simulink model "SOFC_smlkH2"  (R2015b)
settings: Solver=ode113  SolverMode=SingleTasking  StartTime=0.0  StopTime=1000  MaxStep=1  MinStep=0.00001  RelTol=1e-3
values from neighbouring files (symbols this model uses):
  A_an = 1.05e-05    [SOFC_CH4data.m]    (also in SOFC_H2data.m)
  A_cat = 2.38e-05    [SOFC_CH4data.m]    (also in SOFC_H2data.m)
  A_cell = 180    [SOFC_begin.m]
  A_el = 0.03 / T    [SOFC_CH4data.m]    (also in SOFC_H2data.m)
  B_an = -1150    [SOFC_CH4data.m]    (also in SOFC_H2data.m)
  B_cat = 1200    [SOFC_CH4data.m]    (also in SOFC_H2data.m)
  B_el = 10300    [SOFC_CH4data.m]    (also in SOFC_H2data.m)
  c_cw = 4.18e03    (= 4180)    [SOFC_CH4data.m]    (also in SOFC_H2data.m)
  C_th = 500e03    (= 500000)    [SOFC_CH4data.m]    (also in SOFC_H2data.m)
  E_act_an = 75e03    (= 75000)    [SOFC_CH4data.m]    (also in SOFC_H2data.m)
  E_act_cat = 96e03    (= 96000)    [SOFC_CH4data.m]    (also in SOFC_H2data.m)
  eta_ACDC = 0.90    (= 0.9)    [SOFC_CH4data.m]    (also in SOFC_H2data.m = 0.95)
  eta_hx = 0.90    (= 0.9)    [SOFC_CH4data.m]    (also in SOFC_H2data.m = 0.92)
  F = 96485    [SOFC_begin.m]
  F_airsplit = 2.0    (= 2)    [SOFC_CH4data.m]    (also in SOFC_H2data.m = 1.1)
  gamma_an = 5.5e4    (= 55000)    [SOFC_CH4data.m]    (also in SOFC_H2data.m)
  gamma_cat = 7.0e4    (= 70000)    [SOFC_CH4data.m]    (also in SOFC_H2data.m)
  h_airc = gamma_air * R * T / (gamma_air - 1) * ((1 / beta_c)^     ((gamma_air - 1) / gamma_air) - 1) / eta_c    [SOFC_CH4data.m]    (also in SOFC_H2data.m)
  h_airpc = (h_aircomb - h_airexh) / 1000 * M_air    [SOFC_CH4data.m]    (also in SOFC_H2data.m)
  h_airph = (hairph_out - hairph_in) * M_air / eta_ph    [SOFC_H2data.m]
  h_Arpc = (h_Arcomb - h_Arexh) / 1000 * M_Ar    [SOFC_CH4data.m]    (also in SOFC_H2data.m)
  h_CO2pc = (h_CO2comb - h_CO2exh) / 1000 * M_CO2    [SOFC_CH4data.m]    (also in SOFC_H2data.m)
  h_cond = 500    [SOFC_CH4data.m]    (also in SOFC_H2data.m)
  h_conv = 0.1    [SOFC_CH4data.m]    (also in SOFC_H2data.m)
  h_H2c = gamma_H2 * R * T / (gamma_H2 - 1) * ((1 / beta_c)^     ((gamma_H2 - 1) / gamma_H2) - 1) / eta_c    [SOFC_H2data.m]
  h_H2Opc = C_H2Ocomb * (Tcomb - Texh) / 1000 * M_H2O    [SOFC_CH4data.m]    (also in SOFC_H2data.m)
  h_H2Opcvap = WaterEnthalpyVaporization (pcomb/101325, Texh)    [SOFC_CH4data.m]    (also in SOFC_H2data.m)
  h_H2ph = (C_H2phout * TH2out - hH2ph_in) * M_H2 / eta_ph    [SOFC_H2data.m]
  h_N2pc = (h_N2comb - h_N2exh) / 1000 * M_N2    [SOFC_CH4data.m]    (also in SOFC_H2data.m)
  h_O2pc = (h_O2comb - h_O2exh) / 1000 * M_O2    [SOFC_CH4data.m]    (also in SOFC_H2data.m)
  i_max = 0.88    [SOFC_CH4data.m]    (also in SOFC_H2data.m)
  K_H2 = 8.34e-01    (= 0.834)    [SOFC_CH4data.m]    (also in SOFC_H2data.m)
  K_H2O = 2.81e-01    (= 0.281)    [SOFC_CH4data.m]    (also in SOFC_H2data.m)
  K_O2 = 2.52e-00    (= 2.52)    [SOFC_CH4data.m]    (also in SOFC_H2data.m)
  K_r = N_cell / (4 * F)    [SOFC_CH4data.m]    (also in SOFC_H2data.m)
  Kr = I * K_r    [SOFC_H2data.m]
  lambda = 9.15    [SOFC_begin.m]
  m_cw = 0.25000    (= 0.25)    [SOFC_CH4data.m]    (also in SOFC_H2data.m)
  N_cell = 38    [SOFC_begin.m]
  p_atm = 1.01325e05    (= 101325)    [SOFC_begin.m]
  P_gamma = 190.0    (= 190)    [SOFC_CH4data.m]    (also in SOFC_H2data.m = 100)
  p_H20 = pp_fin(6) / 101325    [SOFC_CH4data.m]    (also in SOFC_H2data.m = y_H2in * p_an / 101325)
  p_H2O0 = pp_fin(7) / 101325    [SOFC_CH4data.m]    (also in SOFC_H2data.m = y_H2Oin * p_an / 101325)
  p_O20 = pp_ain(5) / 101325    [SOFC_CH4data.m]    (also in SOFC_H2data.m = x_O2in * p_cat / 101325)
  Q_gamma = 0.0    (= 0)    [SOFC_CH4data.m]    (also in SOFC_H2data.m = 30)
  R = P_SOFC ./ (P_SOFC ./ etae_aux .* etat)    [SOFC_begin.m]
  R_th = 0.0817    [SOFC_CH4data.m]    (also in SOFC_H2data.m)
  T = 750 + 273.15    (= 1023.15)    [SOFC_begin.m]
  T0 = T_a    [SOFC_CH4data.m]    (also in SOFC_H2data.m)
  T_a = 25    [SOFC_begin.m]
  t_an = 0.0545    [SOFC_CH4data.m]    (also in SOFC_H2data.m)
  t_cat = 0.004    [SOFC_CH4data.m]    (also in SOFC_H2data.m)
  T_cwin = 20 + 0    (= 20)    [SOFC_CH4data.m]    (also in SOFC_H2data.m)
  T_des = T - 273.15    [SOFC_CH4data.m]    (also in SOFC_H2data.m)
  t_el = 0.0005    [SOFC_CH4data.m]    (also in SOFC_H2data.m)
  tau_H2 = 26.1    [SOFC_CH4data.m]    (also in SOFC_H2data.m)
  tau_H2O = 78.30    (= 78.3)    [SOFC_CH4data.m]    (also in SOFC_H2data.m)
  tau_hx = 15.0    (= 15)    [SOFC_CH4data.m]    (also in SOFC_H2data.m)
  tau_O2 = 2.91    [SOFC_CH4data.m]    (also in SOFC_H2data.m)
  tau_ph = 5.00    (= 5)    [SOFC_CH4data.m]    (also in SOFC_H2data.m)
  tau_th = C_th * R_th    (= 40850)    [SOFC_CH4data.m]    (also in SOFC_H2data.m)
  theta = 0.910    (= 0.91)    [SOFC_CH4data.m]    (also in SOFC_H2data.m)
  U = polyval(polU, n_CH4in(1))    [SOFC_CH4data.m]    (also in SOFC_H2data.m = polyval(polU, n_H2in(1)))
  V_tn = 1.48    [SOFC_CH4data.m]    (also in SOFC_H2data.m)
  x_Ar = 0.0092    [SOFC_begin.m]
  x_CO2 = 0.0004    [SOFC_begin.m]
  x_H2O = 0.0103    [SOFC_begin.m]
  x_H2Ovap = WaterSaturationPressure (Texh) / (pcomb/101325)    [SOFC_CH4data.m]    (also in SOFC_H2data.m)
  x_N2 = 0.7728    [SOFC_begin.m]
  x_O2 = 0.2073    [SOFC_begin.m]
  xi4 = nn_fout(6) * eta_comb    [SOFC_CH4data.m]    (also in SOFC_H2data.m = n_H2out * eta_comb)
  y_H2in = 0.995    [SOFC_H2data.m]
  y_H2Oin = 1 - y_H2in    (= 0.005)    [SOFC_H2data.m]
undefined symbols (not defined in the file or in its folder): magnitude
settings Model: Creator=gapaolo  LastModifiedBy=gapaolo
settings DataIOCC: SaveFormat=Array
settings OptimizationCC: BlockReduction=off  BooleanDataType=off
settings DebuggingCC: AlgebraicLoopMsg=none  SaveWithParameterizedLinksMsg=none  UnderspecifiedInitializationDetection=Classic  MergeDetectMultiDrivingBlocksExec=none  SignalResolutionControl=TryResolveAllWithWarning
settings HardwareCC: ProdBitPerPointer=32  ProdLargestAtomicFloat=None  ProdIntDivRoundTo=Undefined  ProdEndianess=Unspecified  ProdWordSize=32  ProdHWDeviceType=32-bit Generic  TargetUnknown=on
settings GRTTargetCC: GeneratePreprocessorConditionals=Disable all
settings ConfigComp: CovModelRefEnable=Off  CovSFcnEnable=off

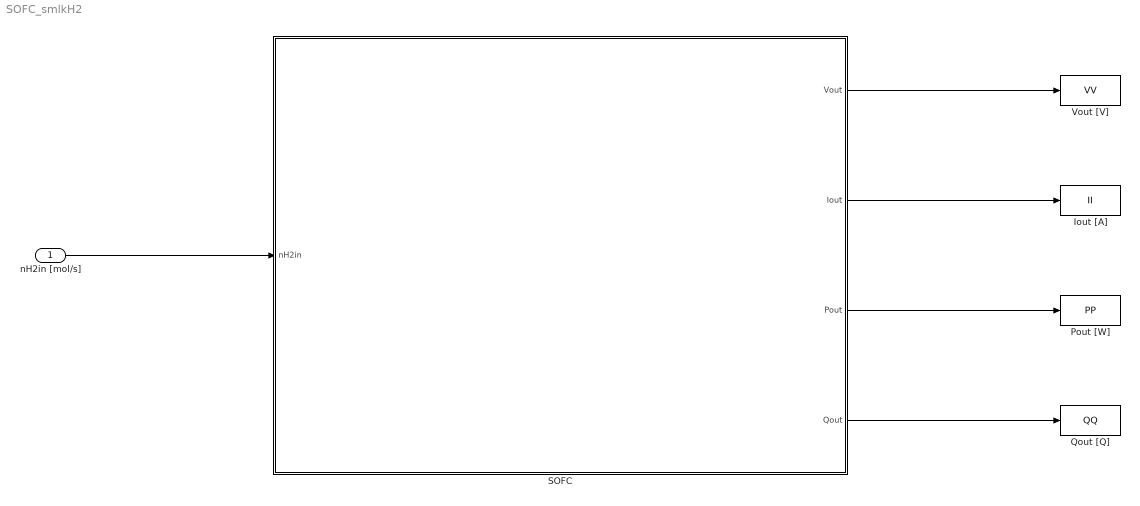
== system SOFC_smlkH2 ==
  nH2in [mol/s] : Inport
  Iout [A] : ToWorkspace  VariableName=II  SaveFormat=Timeseries  SampleTime=-1
  Pout [W] : ToWorkspace  VariableName=PP  SaveFormat=Timeseries  SampleTime=-1
  Qout [Q] : ToWorkspace  VariableName=QQ  SaveFormat=Timeseries  SampleTime=-1
  SOFC : Subsystem
  Vout [V] : ToWorkspace  VariableName=VV  SaveFormat=Timeseries  SampleTime=-1
  wires:
  nH2in [mol/s]/1 -> SOFC/1(nH2in)
  SOFC/1(Vout) -> Vout [V]/1
  SOFC/2(Iout) -> Iout [A]/1
  SOFC/3(Pout) -> Pout [W]/1
  SOFC/4(Qout) -> Qout [Q]/1

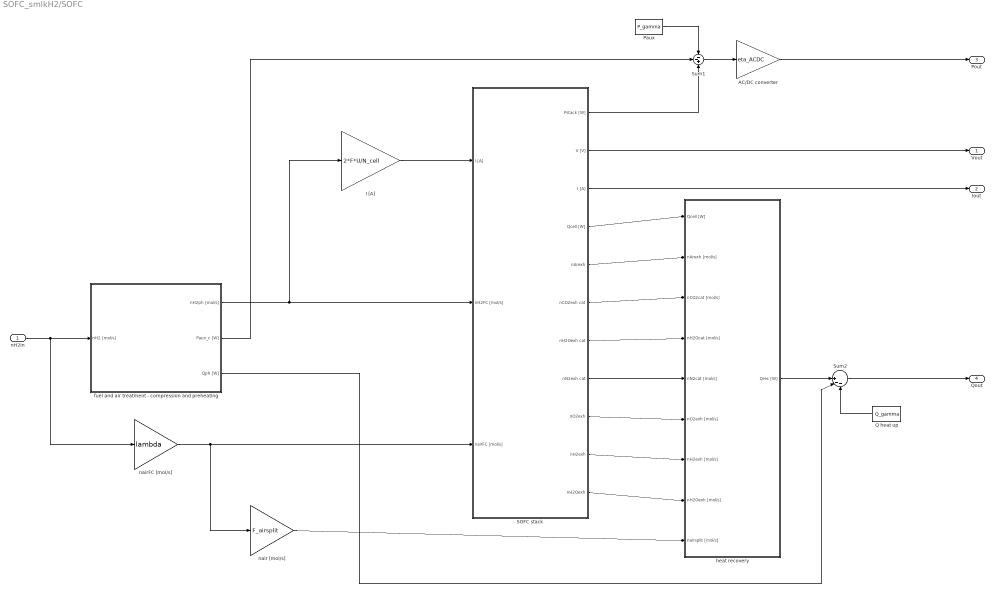
== system SOFC_smlkH2/SOFC ==
  nH2in : Inport
  AC/DC converter : Gain  Gain=eta_ACDC
  I [A] : Gain  Gain=2*F*U/N_cell
  Paux : Constant  Value=P_gamma
  Q heat up : Constant  Value=Q_gamma
  SOFC stack : Subsystem
  Sum1 : Sum  Inputs=--+
  Sum2 : Sum  Inputs=||+--
  fuel and air treatment - compression and preheating : Subsystem
  heat recovery : Subsystem
  nair [mol/s] : Gain  Gain=F_airsplit
  nairFC [mol/s] : Gain  Gain=lambda
  Vout : Outport
  Iout : Outport  Port=2
  Pout : Outport  Port=3
  Qout : Outport  Port=4
  wires:
  nH2in/1 -> fuel and air treatment - compression and preheating/1(nH2 [mol/s]), nairFC [mol/s]/1
  fuel and air treatment - compression and preheating/1(nH2ph [mol/s]) -> I [A]/1, SOFC stack/2(nH2FC [mol/s])
  I [A]/1 -> SOFC stack/1(I [A])
  nairFC [mol/s]/1 -> nair [mol/s]/1, SOFC stack/3(nairFC [mol/s])
  SOFC stack/4(Qcell [W]) -> heat recovery/1(Qcell [W])
  SOFC stack/5(nArexh) -> heat recovery/2(nArexh [mol/s])
  SOFC stack/6(nCO2exh cat) -> heat recovery/3(nCO2cat [mol/s])
  SOFC stack/7(nH2Oexh cat) -> heat recovery/4(nH2Ocat [mol/s])
  SOFC stack/8(nN2exh cat) -> heat recovery/5(nN2cat [mol/s])
  SOFC stack/9(nO2exh) -> heat recovery/6(nO2exh [mol/s])
  nair [mol/s]/1 -> heat recovery/9(nairsplit [mol/s])
  SOFC stack/2(V [V]) -> Vout/1
  SOFC stack/3("I [A] ") -> Iout/1
  Sum1/1 -> AC/DC converter/1
  SOFC stack/1(Pstack [W]) -> Sum1/3
  fuel and air treatment - compression and preheating/2(Paux_c [W]) -> Sum1/2
  Paux/1 -> Sum1/1
  heat recovery/1(Qrec [W]) -> Sum2/1
  Sum2/1 -> Qout/1
  AC/DC converter/1 -> Pout/1
  fuel and air treatment - compression and preheating/3(Qph [W]) -> Sum2/2
  Q heat up/1 -> Sum2/3
  SOFC stack/10(nH2exh) -> heat recovery/7(nH2exh [mol/s])
  SOFC stack/11(nH2Oexh) -> heat recovery/8(nH2Oexh [mol/s])

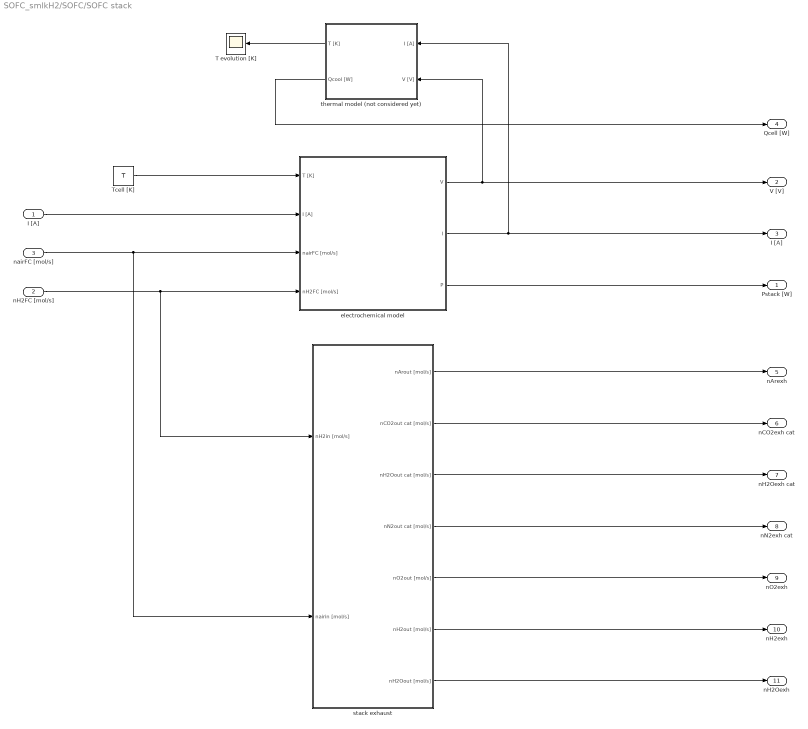
== system SOFC_smlkH2/SOFC/SOFC stack ==
  I [A] : Inport
  nH2FC [mol/s] : Inport  Port=2
  nairFC [mol/s] : Inport  Port=3
  T evolution [K] : Scope
  Tcell [K] : Constant  Value=T
  electrochemical model : Subsystem
  stack exhaust : Subsystem
  thermal model (not considered yet) : Subsystem
  Pstack [W] : Outport
  V [V] : Outport  Port=2
  "I [A] " : Outport  Port=3
  Qcell [W] : Outport  Port=4
  nArexh : Outport  Port=5
  nCO2exh cat : Outport  Port=6
  nH2Oexh cat : Outport  Port=7
  nN2exh cat : Outport  Port=8
  nO2exh : Outport  Port=9
  nH2exh : Outport  Port=10
  nH2Oexh : Outport  Port=11
  wires:
  I [A]/1 -> electrochemical model/2(I [A])
  nairFC [mol/s]/1 -> stack exhaust/2(nairin [mol/s]), electrochemical model/3(nairFC [mol/s])
  nH2FC [mol/s]/1 -> stack exhaust/1(nH2in [mol/s]), electrochemical model/4(nH2FC [mol/s])
  electrochemical model/1(V) -> thermal model (not considered yet)/2(V [V]), V [V]/1
  electrochemical model/2(I) -> thermal model (not considered yet)/1(I [A]), "I [A] "/1
  thermal model (not considered yet)/1(T [K]) -> T evolution [K]/1
  electrochemical model/3(P) -> Pstack [W]/1
  Tcell [K]/1 -> electrochemical model/1(T [K])
  thermal model (not considered yet)/2(Qcool [W]) -> Qcell [W]/1
  stack exhaust/7(nH2Oout [mol/s]) -> nH2Oexh/1
  stack exhaust/5(nO2out [mol/s]) -> nO2exh/1
  stack exhaust/4(nN2out cat [mol/s]) -> nN2exh cat/1
  stack exhaust/3(nH2Oout cat [mol/s]) -> nH2Oexh cat/1
  stack exhaust/2(nCO2out cat [mol/s]) -> nCO2exh cat/1
  stack exhaust/1(nArout [mol/s]) -> nArexh/1
  stack exhaust/6(nH2out [mol/s]) -> nH2exh/1

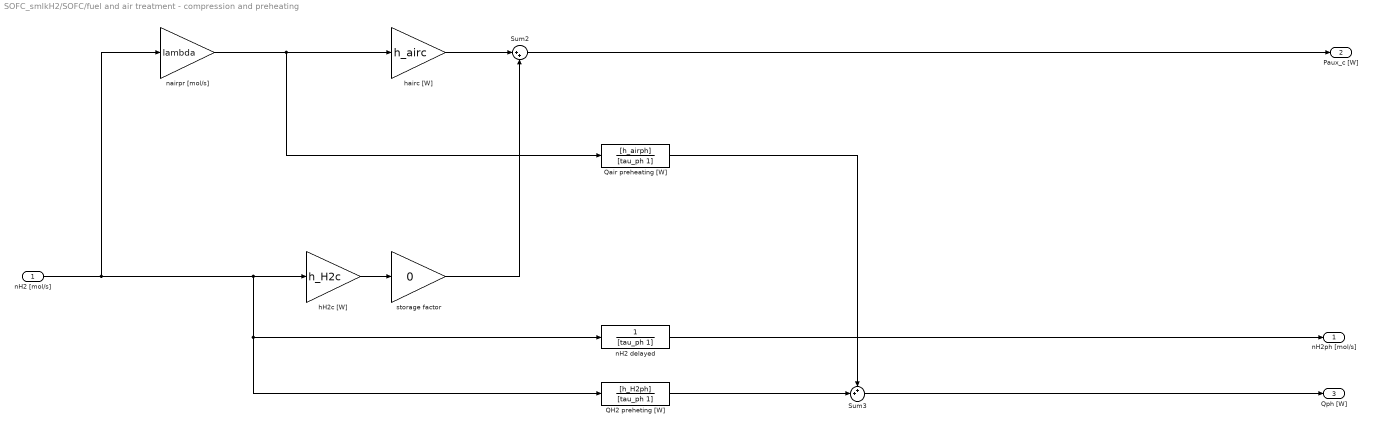
== system SOFC_smlkH2/SOFC/fuel and air treatment - compression and preheating ==
  nH2 [mol/s] : Inport
  QH2 preheting [W] : TransferFcn  Numerator=[h_H2ph]  Denominator=[tau_ph 1]
  Qair preheating [W] : TransferFcn  Numerator=[h_airph]  Denominator=[tau_ph 1]
  Sum2 : Sum  Inputs=|++
  Sum3 : Sum  Inputs=++|
  hH2c [W] : Gain  Gain=h_H2c
  hairc [W] : Gain  Gain=h_airc
  nH2 delayed : TransferFcn  Denominator=[tau_ph 1]
  nairpr [mol/s] : Gain  Gain=lambda
  storage factor : Gain  Gain=0
  nH2ph [mol/s] : Outport
  Paux_c [W] : Outport  Port=2
  Qph [W] : Outport  Port=3
  wires:
  nH2 [mol/s]/1 -> hH2c [W]/1, nH2 delayed/1, QH2 preheting [W]/1, nairpr [mol/s]/1
  nairpr [mol/s]/1 -> Qair preheating [W]/1, hairc [W]/1
  hairc [W]/1 -> Sum2/1
  hH2c [W]/1 -> storage factor/1
  Sum2/1 -> Paux_c [W]/1
  Sum3/1 -> Qph [W]/1
  Qair preheating [W]/1 -> Sum3/1
  QH2 preheting [W]/1 -> Sum3/2
  nH2 delayed/1 -> nH2ph [mol/s]/1
  storage factor/1 -> Sum2/2

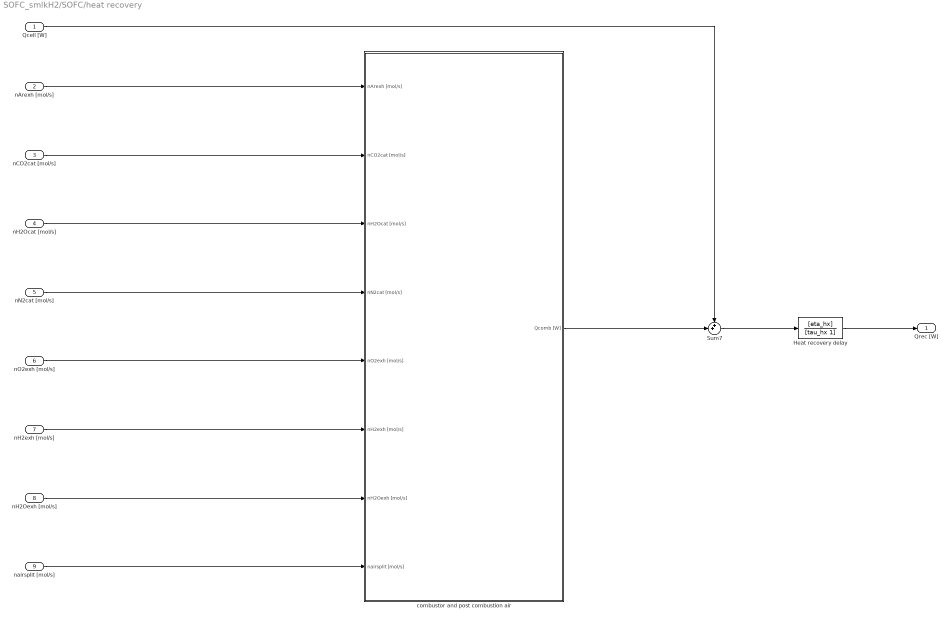
== system SOFC_smlkH2/SOFC/heat recovery ==
  Qcell [W] : Inport
  nArexh [mol/s] : Inport  Port=2
  nCO2cat [mol/s] : Inport  Port=3
  nH2Ocat [mol/s] : Inport  Port=4
  nN2cat [mol/s] : Inport  Port=5
  nO2exh [mol/s] : Inport  Port=6
  nH2exh [mol/s] : Inport  Port=7
  nH2Oexh [mol/s] : Inport  Port=8
  nairsplit [mol/s] : Inport  Port=9
  Heat recovery delay : TransferFcn  Numerator=[eta_hx]  Denominator=[tau_hx 1]
  Sum7 : Sum  Inputs=++|
  combustor and post combustion air : Subsystem
  Qrec [W] : Outport
  wires:
  Heat recovery delay/1 -> Qrec [W]/1
  nArexh [mol/s]/1 -> combustor and post combustion air/1(nArexh [mol/s])
  nCO2cat [mol/s]/1 -> combustor and post combustion air/2(nCO2cat [mol/s])
  nH2Ocat [mol/s]/1 -> combustor and post combustion air/3(nH2Ocat [mol/s])
  nN2cat [mol/s]/1 -> combustor and post combustion air/4(nN2cat [mol/s])
  nO2exh [mol/s]/1 -> combustor and post combustion air/5(nO2exh [mol/s])
  nH2exh [mol/s]/1 -> combustor and post combustion air/6(nH2exh [mol/s])
  nH2Oexh [mol/s]/1 -> combustor and post combustion air/7(nH2Oexh [mol/s])
  combustor and post combustion air/1(Qcomb [W]) -> Sum7/2
  Sum7/1 -> Heat recovery delay/1
  Qcell [W]/1 -> Sum7/1
  nairsplit [mol/s]/1 -> combustor and post combustion air/8(nairsplit [mol/s])

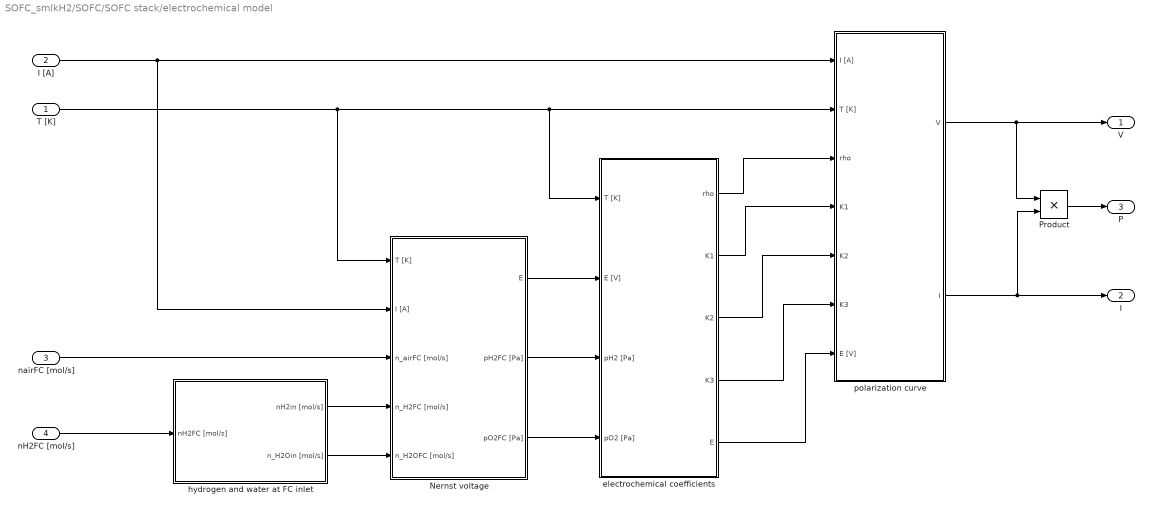
== system SOFC_smlkH2/SOFC/SOFC stack/electrochemical model ==
  T [K] : Inport
  I [A] : Inport  Port=2
  nairFC [mol/s] : Inport  Port=3
  nH2FC [mol/s] : Inport  Port=4
  Nernst voltage : Subsystem
  Product : Product
  electrochemical coefficients : Subsystem
  hydrogen and water at FC inlet : Subsystem
  polarization curve : Subsystem
  V : Outport
  I : Outport  Port=2
  P : Outport  Port=3
  wires:
  hydrogen and water at FC inlet/1(nH2in [mol/s]) -> Nernst voltage/4(n_H2FC [mol/s])
  nairFC [mol/s]/1 -> Nernst voltage/3(n_airFC [mol/s])
  T [K]/1 -> Nernst voltage/1(T [K]), polarization curve/2(T [K]), electrochemical coefficients/1(T [K])
  hydrogen and water at FC inlet/2(n_H2Oin [mol/s]) -> Nernst voltage/5(n_H2OFC [mol/s])
  nH2FC [mol/s]/1 -> hydrogen and water at FC inlet/1(nH2FC [mol/s])
  I [A]/1 -> Nernst voltage/2(I [A]), polarization curve/1("I [A] ")
  Nernst voltage/2(pH2FC [Pa]) -> electrochemical coefficients/3("pH2 [Pa] ")
  Nernst voltage/3(pO2FC [Pa]) -> electrochemical coefficients/4(pO2 [Pa])
  Nernst voltage/1(E) -> electrochemical coefficients/2(E [V])
  electrochemical coefficients/1(rho) -> polarization curve/3(rho)
  electrochemical coefficients/2(K1) -> polarization curve/4(K1)
  electrochemical coefficients/3(K2) -> polarization curve/5(K2)
  electrochemical coefficients/4(K3) -> polarization curve/6(K3)
  electrochemical coefficients/5(E) -> polarization curve/7(E [V])
  polarization curve/2(I) -> Product/2, I/1
  polarization curve/1(V) -> Product/1, V/1
  Product/1 -> P/1

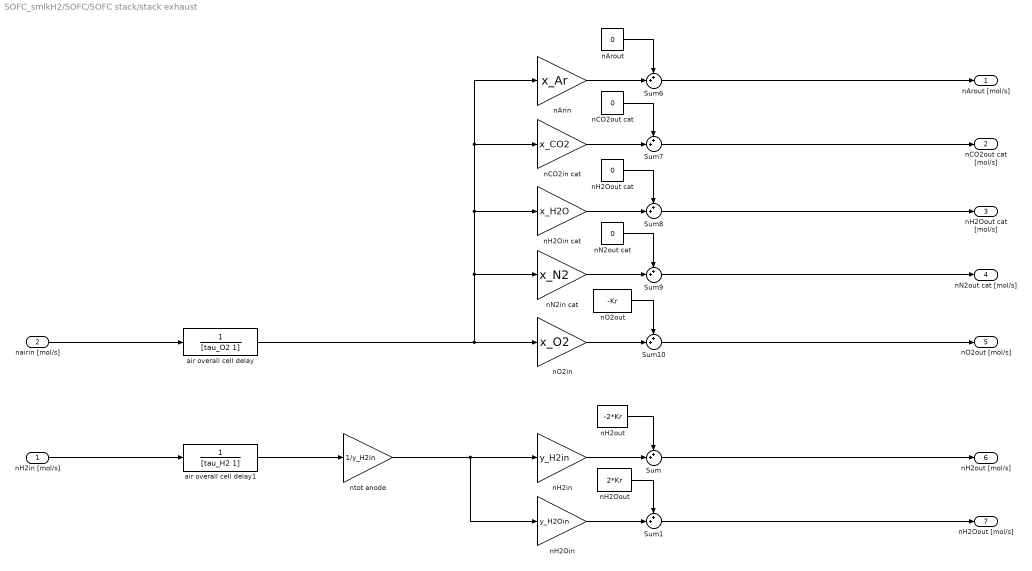
== system SOFC_smlkH2/SOFC/SOFC stack/stack exhaust ==
  nH2in [mol/s] : Inport
  nairin [mol/s] : Inport  Port=2
  Sum{,1,6..10} (7 alike) : Sum  Inputs=++|
  air overall cell delay : TransferFcn  Denominator=[tau_O2 1]  ContinuousStateAttributes='p_O2'
  air overall cell delay1 : TransferFcn  Denominator=[tau_H2 1]  ContinuousStateAttributes='p_O2'
  nArin : Gain  Gain=x_Ar
  nArout : Constant  Value=0
  nCO2in cat : Gain  Gain=x_CO2
  nCO2out cat : Constant  Value=0
  nH2Oin : Gain  Gain=y_H2Oin
  nH2Oin cat : Gain  Gain=x_H2O
  nH2Oout : Constant  Value=2*Kr
  nH2Oout cat : Constant  Value=0
  nH2in : Gain  Gain=y_H2in
  nH2out : Constant  Value=-2*Kr
  nN2in cat : Gain  Gain=x_N2
  nN2out cat : Constant  Value=0
  nO2in : Gain  Gain=x_O2
  nO2out : Constant  Value=-Kr
  ntot anode : Gain  Gain=1/y_H2in
  nArout [mol/s] : Outport
  nCO2out cat [mol/s] : Outport  Port=2
  nH2Oout cat [mol/s] : Outport  Port=3
  nN2out cat [mol/s] : Outport  Port=4
  nO2out [mol/s] : Outport  Port=5
  nH2out [mol/s] : Outport  Port=6
  nH2Oout [mol/s] : Outport  Port=7
  wires:
  nH2in [mol/s]/1 -> air overall cell delay1/1
  nairin [mol/s]/1 -> air overall cell delay/1
  air overall cell delay1/1 -> ntot anode/1
  nH2in/1 -> Sum/2
  nH2out/1 -> Sum/1
  nH2Oin/1 -> Sum1/2
  nH2Oout/1 -> Sum1/1
  nArin/1 -> Sum6/2
  nArout/1 -> Sum6/1
  nCO2in cat/1 -> Sum7/2
  nCO2out cat/1 -> Sum7/1
  nH2Oin cat/1 -> Sum8/2
  nH2Oout cat/1 -> Sum8/1
  nN2in cat/1 -> Sum9/2
  nN2out cat/1 -> Sum9/1
  nO2in/1 -> Sum10/2
  nO2out/1 -> Sum10/1
  air overall cell delay/1 -> nH2Oin cat/1, nCO2in cat/1, nArin/1, nN2in cat/1, nO2in/1
  Sum6/1 -> nArout [mol/s]/1
  Sum7/1 -> nCO2out cat [mol/s]/1
  Sum8/1 -> nH2Oout cat [mol/s]/1
  Sum9/1 -> nN2out cat [mol/s]/1
  Sum10/1 -> nO2out [mol/s]/1
  Sum1/1 -> nH2Oout [mol/s]/1
  Sum/1 -> nH2out [mol/s]/1
  ntot anode/1 -> nH2Oin/1, nH2in/1

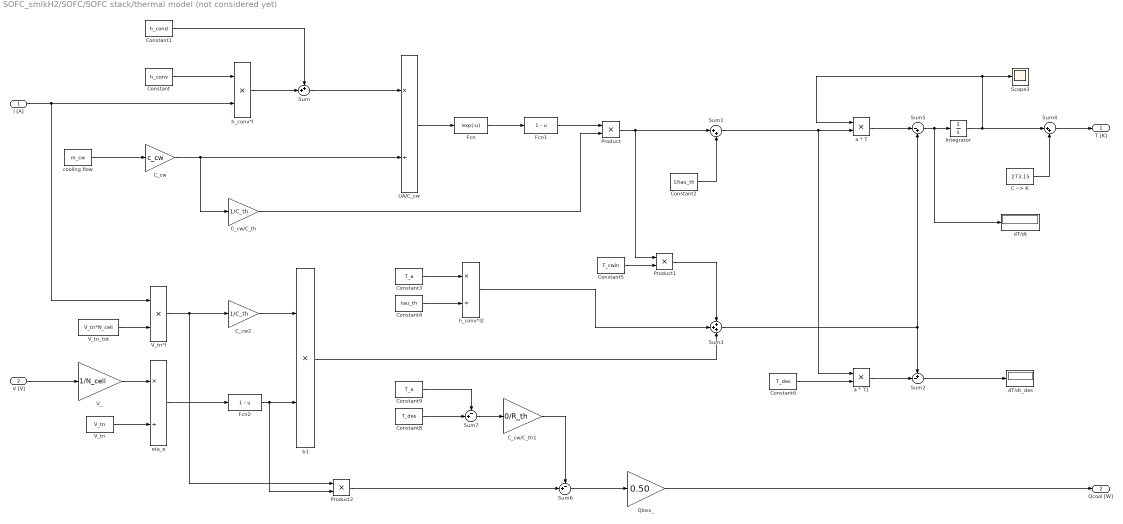
== system SOFC_smlkH2/SOFC/SOFC stack/thermal model (not considered yet) ==
  I [A] : Inport
  V [V] : Inport  Port=2
  C --> K : Constant  Value=273.15
  C_cw : Gain  Gain=c_cw
  C_cw/C_th : Gain  Gain=1/C_th
  C_cw/C_th1 : Gain  Gain=0/R_th
  C_cw2 : Gain  Gain=1/C_th
  Constant : Constant  Value=h_conv
  Constant1 : Constant  Value=h_cond
  Constant2 : Constant  Value=1/tau_th
  Constant3 : Constant  Value=T_a
  Constant4 : Constant  Value=tau_th
  Constant5 : Constant  Value=T_cwin
  Constant6 : Constant  Value=T_des
  Constant8 : Constant  Value=T_des
  Constant9 : Constant  Value=T_a
  Fcn : Fcn  Expr=exp(-u)
  Fcn1 : Fcn  Expr=1 - u
  Fcn2 : Fcn  Expr=1 - u
  Integrator : Integrator  InitialCondition=T0  AbsoluteTolerance=1e-6
  Product : Product
  Product1 : Product
  Product2 : Product
  Qloss_ : Gain  Gain=0.50
  Scope3 : Scope
  Sum : Sum  Inputs=++|
  Sum1 : Sum  Inputs=|++
  Sum2 : Sum  Inputs=+-|
  Sum3 : Sum  Inputs=+++
  Sum4 : Sum  Inputs=|++
  Sum5 : Sum  Inputs=|-+
  Sum6 : Sum  Inputs=-+|
  Sum7 : Sum  Inputs=-+|
  UA/C_cw : Product  Inputs=*/
  V_ : Gain  Gain=1/N_cell
  V_tn : Constant  Value=V_tn
  V_tn*I : Product
  V_tn_tot : Constant  Value=V_tn*N_cell
  a * T : Product
  a * T1 : Product
  b1 : Product
  cooling flow : Constant  Value=m_cw
  dT/dt : Display
  dT/dt_des : Display
  eta_e : Product  Inputs=*/
  h_conv*I : Product
  h_conv*I2 : Product  Inputs=*/
  T [K] : Outport
  Qcool [W] : Outport  Port=2
  wires:
  V_tn_tot/1 -> V_tn*I/2
  eta_e/1 -> Fcn2/1
  V_tn/1 -> eta_e/2
  V_/1 -> eta_e/1
  b1/1 -> Sum3/3
  h_conv*I2/1 -> Sum3/2
  Product1/1 -> Sum3/1
  Constant5/1 -> Product1/2
  Constant4/1 -> h_conv*I2/2
  Constant3/1 -> h_conv*I2/1
  C_cw2/1 -> b1/1
  V [V]/1 -> V_/1
  Constant2/1 -> Sum1/2
  Product/1 -> Sum1/1, Product1/1
  C_cw/C_th/1 -> Product/2
  Fcn1/1 -> Product/1
  C_cw/1 -> C_cw/C_th/1, UA/C_cw/2
  Fcn/1 -> Fcn1/1
  UA/C_cw/1 -> Fcn/1
  cooling flow/1 -> C_cw/1
  Sum/1 -> UA/C_cw/1
  Constant1/1 -> Sum/1
  h_conv*I/1 -> Sum/2
  Constant/1 -> h_conv*I/1
  I [A]/1 -> h_conv*I/2, V_tn*I/1
  Integrator/1 -> Sum4/1, a * T/1, Scope3/1
  a * T/1 -> Sum5/1
  Sum3/1 -> Sum5/2, Sum2/1
  Sum1/1 -> a * T1/1, a * T/2
  Constant6/1 -> a * T1/2
  a * T1/1 -> Sum2/2
  Sum2/1 -> dT/dt_des/1
  C --> K/1 -> Sum4/2
  Sum4/1 -> T [K]/1
  Product2/1 -> Sum6/2
  Constant8/1 -> Sum7/2
  Constant9/1 -> Sum7/1
  Sum7/1 -> C_cw/C_th1/1
  C_cw/C_th1/1 -> Sum6/1
  V_tn*I/1 -> Product2/1, C_cw2/1
  Fcn2/1 -> Product2/2, b1/2
  Sum5/1 -> dT/dt/1, Integrator/1
  Sum6/1 -> Qloss_/1
  Qloss_/1 -> Qcool [W]/1

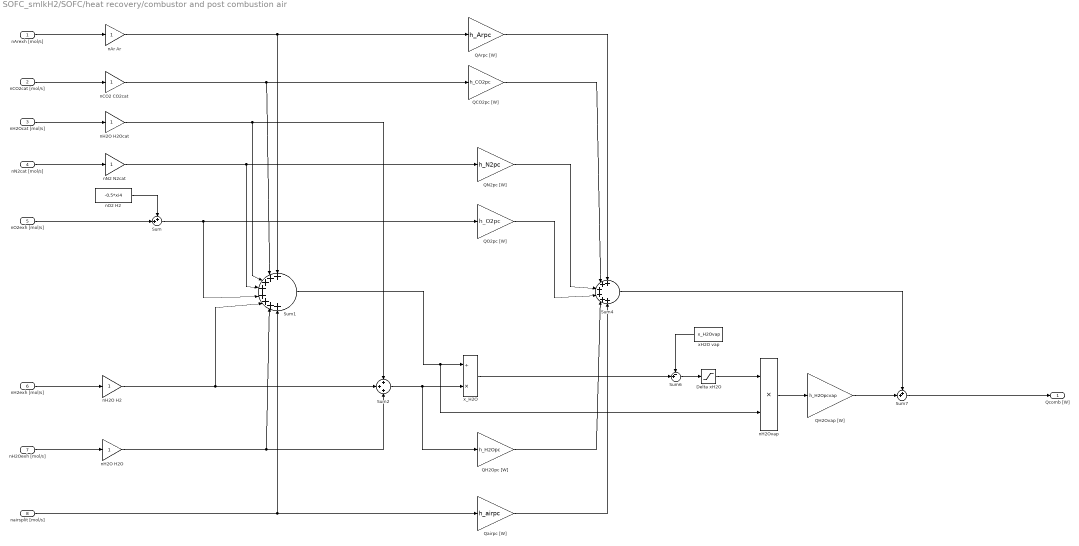
== system SOFC_smlkH2/SOFC/heat recovery/combustor and post combustion air ==
  nArexh [mol/s] : Inport
  nCO2cat [mol/s] : Inport  Port=2
  nH2Ocat [mol/s] : Inport  Port=3
  nN2cat [mol/s] : Inport  Port=4
  nO2exh [mol/s] : Inport  Port=5
  nH2exh [mol/s] : Inport  Port=6
  nH2Oexh [mol/s] : Inport  Port=7
  nairsplit [mol/s] : Inport  Port=8
  Delta xH2O : Saturate  UpperLimit=1  LowerLimit=0
  QArpc [W] : Gain  Gain=h_Arpc
  QCO2pc [W] : Gain  Gain=h_CO2pc
  QH2Opc [W] : Gain  Gain=h_H2Opc
  QH2Ovap [W] : Gain  Gain=h_H2Opcvap
  QN2pc [W] : Gain  Gain=h_N2pc
  QO2pc [W] : Gain  Gain=h_O2pc
  Qairpc [W] : Gain  Gain=h_airpc
  Sum : Sum  Inputs=++|
  Sum1 : Sum  Inputs=++++++++
  Sum2 : Sum  Inputs=+++
  Sum4 : Sum  Inputs=++++++
  Sum6 : Sum  Inputs=-+|
  Sum7 : Sum  Inputs=++|
  nAr Ar : Gain
  nCO2 CO2cat : Gain
  nH2O H2 : Gain
  nH2O H2O : Gain
  nH2O H2Ocat : Gain
  nH2Ovap : Product  Inputs=**
  nN2 N2cat : Gain
  nO2 H2 : Constant  Value=-0.5*xi4
  xH2O vap : Constant  Value=x_H2Ovap
  x_H2O : Product  Inputs=/*
  Qcomb [W] : Outport
  wires:
  Delta xH2O/1 -> nH2Ovap/1
  x_H2O/1 -> Sum6/2
  QArpc [W]/1 -> Sum4/1
  Qairpc [W]/1 -> Sum4/6
  nH2Ovap/1 -> QH2Ovap [W]/1
  Sum6/1 -> Delta xH2O/1
  Sum1/1 -> x_H2O/1, nH2Ovap/2
  xH2O vap/1 -> Sum6/1
  QH2Ovap [W]/1 -> Sum7/2
  Sum7/1 -> Qcomb [W]/1
  nArexh [mol/s]/1 -> nAr Ar/1
  nCO2cat [mol/s]/1 -> nCO2 CO2cat/1
  nH2Ocat [mol/s]/1 -> nH2O H2Ocat/1
  nN2cat [mol/s]/1 -> nN2 N2cat/1
  nO2exh [mol/s]/1 -> Sum/2
  nO2 H2/1 -> Sum/1
  nH2exh [mol/s]/1 -> nH2O H2/1
  nH2Oexh [mol/s]/1 -> nH2O H2O/1
  nairsplit [mol/s]/1 -> Qairpc [W]/1, Sum1/8
  nH2O H2O/1 -> Sum2/3, Sum1/7
  nH2O H2/1 -> Sum1/6, Sum2/2
  Sum/1 -> Sum1/5, QO2pc [W]/1
  nN2 N2cat/1 -> Sum1/4, QN2pc [W]/1
  nCO2 CO2cat/1 -> QCO2pc [W]/1, Sum1/2
  nAr Ar/1 -> QArpc [W]/1, Sum1/1
  nH2O H2Ocat/1 -> Sum2/1, Sum1/3
  Sum2/1 -> x_H2O/2, QH2Opc [W]/1
  Sum4/1 -> Sum7/1
  QH2Opc [W]/1 -> Sum4/5
  QO2pc [W]/1 -> Sum4/4
  QN2pc [W]/1 -> Sum4/3
  QCO2pc [W]/1 -> Sum4/2

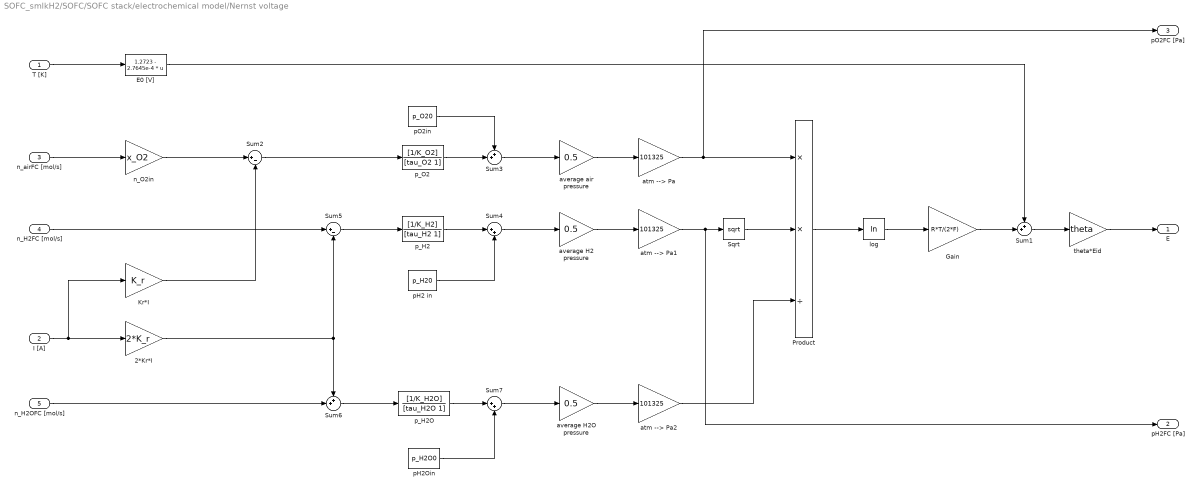
== system SOFC_smlkH2/SOFC/SOFC stack/electrochemical model/Nernst voltage ==
  T [K] : Inport
  I [A] : Inport  Port=2
  n_airFC [mol/s] : Inport  Port=3
  n_H2FC [mol/s] : Inport  Port=4
  n_H2OFC [mol/s] : Inport  Port=5
  2*Kr*I : Gain  Gain=2*K_r
  E0 [V] : Fcn  Expr=1.2723 - 2.7645e-4 * u
  Gain : Gain  Gain=R*T/(2*F)
  Kr*I : Gain  Gain=K_r
  Product : Product  Inputs=**/
  Sqrt : Sqrt  SaturateOnIntegerOverflow=on
  Sum1 : Sum  Inputs=++|
  Sum2 : Sum  Inputs=|+-
  Sum3 : Sum  Inputs=++|
  Sum4 : Sum  Inputs=|++
  Sum5 : Sum  Inputs=|+-
  Sum6 : Sum  Inputs=++|
  Sum7 : Sum  Inputs=|++
  atm --> Pa : Gain  Gain=101325
  atm --> Pa1 : Gain  Gain=101325
  atm --> Pa2 : Gain  Gain=101325
  average H2 pressure : Gain  Gain=0.5
  average H2O pressure : Gain  Gain=0.5
  average air pressure : Gain  Gain=0.5
  log : Math  Operator=log  SaturateOnIntegerOverflow=on
  n_O2in : Gain  Gain=x_O2
  pH2 in : Constant  Value=p_H20
  pH2Oin : Constant  Value=p_H2O0
  pO2in : Constant  Value=p_O20
  p_H2 : TransferFcn  Numerator=[1/K_H2]  Denominator=[tau_H2 1]  ContinuousStateAttributes='p_H2'
  p_H2O : TransferFcn  Numerator=[1/K_H2O]  Denominator=[tau_H2O 1]  ContinuousStateAttributes='p_H2'
  p_O2 : TransferFcn  Numerator=[1/K_O2]  Denominator=[tau_O2 1]  ContinuousStateAttributes='p_O2'
  theta*Eid : Gain  Gain=theta
  E : Outport
  pH2FC [Pa] : Outport  Port=2
  pO2FC [Pa] : Outport  Port=3
  wires:
  n_airFC [mol/s]/1 -> n_O2in/1
  p_H2/1 -> Sum4/1
  p_O2/1 -> Sum3/2
  pH2 in/1 -> Sum4/2
  pO2in/1 -> Sum3/1
  Sum3/1 -> average air pressure/1
  Sum4/1 -> average H2 pressure/1
  p_H2O/1 -> Sum7/1
  pH2Oin/1 -> Sum7/2
  Sqrt/1 -> Product/2
  Gain/1 -> Sum1/2
  E0 [V]/1 -> Sum1/1
  Sum1/1 -> theta*Eid/1
  log/1 -> Gain/1
  Product/1 -> log/1
  theta*Eid/1 -> E/1
  atm --> Pa1/1 -> pH2FC [Pa]/1, Sqrt/1
  atm --> Pa2/1 -> Product/3
  Sum7/1 -> average H2O pressure/1
  atm --> Pa/1 -> pO2FC [Pa]/1, Product/1
  T [K]/1 -> E0 [V]/1
  average air pressure/1 -> atm --> Pa/1
  average H2 pressure/1 -> atm --> Pa1/1
  average H2O pressure/1 -> atm --> Pa2/1
  I [A]/1 -> Kr*I/1, 2*Kr*I/1
  Kr*I/1 -> Sum2/2
  n_O2in/1 -> Sum2/1
  Sum2/1 -> p_O2/1
  Sum5/1 -> p_H2/1
  n_H2FC [mol/s]/1 -> Sum5/1
  2*Kr*I/1 -> Sum6/1, Sum5/2
  n_H2OFC [mol/s]/1 -> Sum6/2
  Sum6/1 -> p_H2O/1

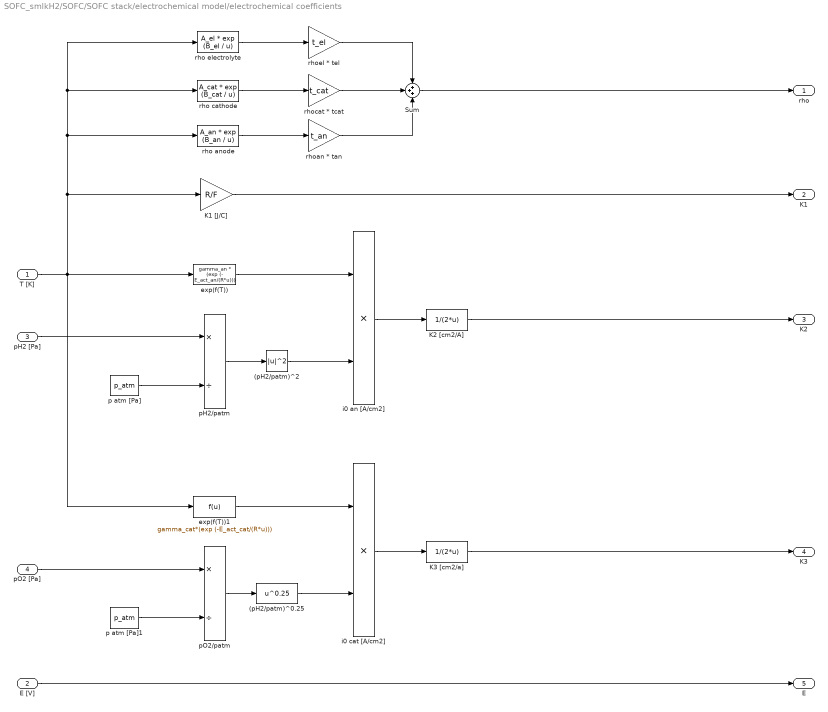
== system SOFC_smlkH2/SOFC/SOFC stack/electrochemical model/electrochemical coefficients ==
  T [K] : Inport
  E [V] : Inport  Port=2
  "pH2 [Pa] " : Inport  Port=3
  pO2 [Pa] : Inport  Port=4
  (pH2/patm)^0.25 : Fcn  Expr=u^0.25
  (pH2/patm)^2 : Math  Operator=magnitude^2  SaturateOnIntegerOverflow=on
  K1 [J/C] : Gain  Gain=R/F
  K2 [cm2/A] : Fcn  Expr=1/(2*u)
  K3 [cm2/a] : Fcn  Expr=1/(2*u)
  Sum : Sum  Inputs=+++
  exp(f(T)) : Fcn  Expr=gamma_an * (exp (- E_act_an/(R*u)))
  exp(f(T))1 : Fcn  Expr=gamma_cat*(exp (-E_act_cat/(R*u)))
  i0 an [A/cm2] : Product
  i0 cat [A/cm2] : Product
  p atm [Pa] : Constant  Value=p_atm
  p atm [Pa]1 : Constant  Value=p_atm
  pH2/patm : Product  Inputs=*/
  pO2/patm : Product  Inputs=*/
  rho anode : Fcn  Expr=A_an * exp (B_an / u)
  rho cathode : Fcn  Expr=A_cat * exp (B_cat / u)
  rho electrolyte : Fcn  Expr=A_el * exp (B_el / u)
  rhoan * tan : Gain  Gain=t_an
  rhocat * tcat : Gain  Gain=t_cat
  rhoel * tel : Gain  Gain=t_el
  rho : Outport
  K1 : Outport  Port=2
  K2 : Outport  Port=3
  K3 : Outport  Port=4
  E : Outport  Port=5
  wires:
  "pH2 [Pa] "/1 -> pH2/patm/1
  p atm [Pa]/1 -> pH2/patm/2
  pH2/patm/1 -> (pH2/patm)^2/1
  T [K]/1 -> rho electrolyte/1, rho cathode/1, rho anode/1, K1 [J/C]/1, exp(f(T))1/1, exp(f(T))/1
  exp(f(T))/1 -> i0 an [A/cm2]/1
  (pH2/patm)^2/1 -> i0 an [A/cm2]/2
  p atm [Pa]1/1 -> pO2/patm/2
  pO2 [Pa]/1 -> pO2/patm/1
  pO2/patm/1 -> (pH2/patm)^0.25/1
  (pH2/patm)^0.25/1 -> i0 cat [A/cm2]/2
  exp(f(T))1/1 -> i0 cat [A/cm2]/1
  i0 an [A/cm2]/1 -> K2 [cm2/A]/1
  i0 cat [A/cm2]/1 -> K3 [cm2/a]/1
  rho electrolyte/1 -> rhoel * tel/1
  rho cathode/1 -> rhocat * tcat/1
  rho anode/1 -> rhoan * tan/1
  rhocat * tcat/1 -> Sum/2
  rhoan * tan/1 -> Sum/3
  rhoel * tel/1 -> Sum/1
  Sum/1 -> rho/1
  K1 [J/C]/1 -> K1/1
  K2 [cm2/A]/1 -> K2/1
  K3 [cm2/a]/1 -> K3/1
  E [V]/1 -> E/1

== system SOFC_smlkH2/SOFC/SOFC stack/electrochemical model/hydrogen and water at FC inlet ==
  nH2FC [mol/s] : Inport
  n anode [mol/s] : Gain  Gain=1/y_H2in
  nH2 [mol/s] : Gain  Gain=y_H2in
  nH2O [mol/s] : Gain  Gain=y_H2Oin
  nH2in [mol/s] : Outport
  n_H2Oin [mol/s] : Outport  Port=2
  wires:
  nH2FC [mol/s]/1 -> n anode [mol/s]/1
  n anode [mol/s]/1 -> nH2O [mol/s]/1, nH2 [mol/s]/1
  nH2O [mol/s]/1 -> n_H2Oin [mol/s]/1
  nH2 [mol/s]/1 -> nH2in [mol/s]/1

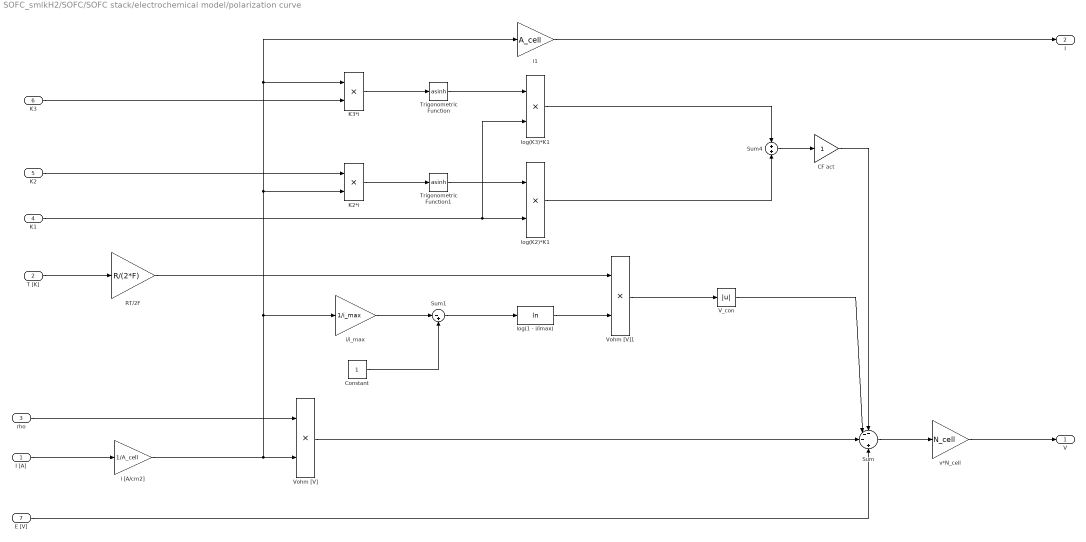
== system SOFC_smlkH2/SOFC/SOFC stack/electrochemical model/polarization curve ==
  "I [A] " : Inport
  T [K] : Inport  Port=2
  rho : Inport  Port=3
  K1 : Inport  Port=4
  K2 : Inport  Port=5
  K3 : Inport  Port=6
  E [V] : Inport  Port=7
  CF act : Gain
  Constant : Constant
  K2*i : Product
  K3*i : Product
  RT/2F : Gain  Gain=R/(2*F)
  Sum : Sum  Inputs=---|+
  Sum1 : Sum  Inputs=|-+
  Sum4 : Sum  Inputs=+|+
  Trigonometric Function : Trigonometry  Operator=asinh
  Trigonometric Function1 : Trigonometry  Operator=asinh
  V_con : Abs
  Vohm [V] : Product
  Vohm [V]1 : Product
  i [A/cm2] : Gain  Gain=1/A_cell
  i/i_max : Gain  Gain=1/i_max
  i1 : Gain  Gain=A_cell
  log(1 - i/imax) : Math  Operator=log  SaturateOnIntegerOverflow=on
  log(K2)*K1 : Product
  log(K3)*K1 : Product
  v*N_cell : Gain  Gain=N_cell
  V : Outport
  I : Outport  Port=2
  wires:
  Vohm [V]/1 -> Sum/3
  v*N_cell/1 -> V/1
  "I [A] "/1 -> i [A/cm2]/1
  Sum/1 -> v*N_cell/1
  Vohm [V]1/1 -> V_con/1
  K2*i/1 -> Trigonometric Function1/1
  K3*i/1 -> Trigonometric Function/1
  Trigonometric Function1/1 -> log(K2)*K1/1
  Trigonometric Function/1 -> log(K3)*K1/1
  log(K2)*K1/1 -> Sum4/2
  log(K3)*K1/1 -> Sum4/1
  Sum4/1 -> CF act/1
  i [A/cm2]/1 -> K3*i/1, i1/1, K2*i/2, i/i_max/1, Vohm [V]/2
  Sum1/1 -> log(1 - i/imax)/1
  log(1 - i/imax)/1 -> Vohm [V]1/2
  i1/1 -> I/1
  V_con/1 -> Sum/2
  E [V]/1 -> Sum/4
  rho/1 -> Vohm [V]/1
  T [K]/1 -> RT/2F/1
  RT/2F/1 -> Vohm [V]1/1
  i/i_max/1 -> Sum1/1
  Constant/1 -> Sum1/2
  K2/1 -> K2*i/1
  K1/1 -> log(K3)*K1/2, log(K2)*K1/2
  K3/1 -> K3*i/2
  CF act/1 -> Sum/1
